simulink model "CusakisME4901delay"  (R2013a)
settings: Solver=ode4  StartTime=0.0  StopTime=inf  FixedStep=0.01  RelTol=1e-3
InitFcn:
  | start_EEVSCube2
  | 
  | %links masses
  | 
  | m=20;%Kg
  | 
  | l=1;%meter
  | 
  | w=0.08;
  | 
  | I=(1/12)*m*(l^2); %moment of inertia
  | 
  | %estimation error
  | 
  | mn=20+m*0.05;
  | In=I+I*0.1;
  | 
  | %controls
  | 
  | a=0.7; %singularity positive gain
  | 
  | %Chaser
  | mb=100;%kg
  | lc=2;%meters
  | lb=lc/2;%meter distance 1joint to CM
  | Ib=(1/12)*mb*(lc^2+lc^2);
  | 
  | %Target
  | 
  | mt=750;%kg target mass
  | lt=1;%meter  side lenght
  | It=(1/6)*(lt^2)*mt;
  | 
  | %Target Initial Conitions
  | 
  | x_t=2;
  | y_t=2;
  | theta_t=0.7853;
  | 
  | Init_t=[x_t;y_t;theta_t;0;0;0];
  | Iinv=pinv(eye(3)*It);
StopFcn:
  | figure(1)
  | subplot(2,1,1)
  | hold on
  | plot(time,kinetic,'g')
  | grid on
  | title('Kinetic Energy vs Time')
  | xlabel('Time')
  | ylabel('Kinetic Energy')
  | hold off
  | 
  | subplot(2,1,2)
  | hold on
  | plot(time,power,'g')
  | grid on
  | title('Power Consumption vs Time')
  | xlabel('Time')
  | ylabel('Power')
  | hold off
  | 
  | chasermapping=[-1,1;-1,-1;1,-1;1,1;-1,1];
  | targetmapping=[1.293,2;2,2.707;2.707,2;2,1.293;1.293,2];
  | 
  | figure(3)
  | hold on
  | plot(EEstate(:,1),EEstate(:,2),'g')
  | plot(targetmapping(:,1),targetmapping(:,2),'r')
  | plot(chasermapping(:,1),chasermapping(:,2),'b')
  | grid on
  | title('End Effector Path')
  | xlabel('X Axis (m)')
  | ylabel('Y Axis (m)')
  | hold off
  | 
  | 
  | figure(4)
  | subplot(2,1,1)
  | hold on
  | plot(time,qqd(:,1),'g')
  | plot(time,qqd(:,2),'r')
  | plot(time,qqd(:,3),'b')
  | grid on
  | title('Theta vs Time')
  | xlabel('Time (sec)')
  | ylabel('Theta (rad)')
  | legend( 'Theta1 ' , ' Theta2 ' , ' Theta3')
  | hold off
  | 
  | subplot(2,1,2)
  | hold on
  | plot(time,qqd(:,4),'g')
  | plot(time,qqd(:,5),'r')
  | plot(time,qqd(:,6),'b')
  | grid on
  | legend( 'Omega1 ' , ' Omega2 ', ' Omega3 ' )
  | title('Omega vs Time')
  | xlabel('Time (sec)')
  | ylabel('Omega (rad/s)')
undefined symbols (not defined in the file): mesh_A, mesh_B, serial
libraries: instrumentlib x5, simulink x3, vrlib x2, dspinverses x1, aerolibanimutils x1
(part 3 of 4)

== matlab function CusakisME4901delay/Differential Kinematics1/Differential Kinematics and singularity avoidance ==
  data: Ve input; qqd input; qd_req output; qd_reqW output; l parameter; a parameter; W output; EE input
function [qd_req,qd_reqW,W]   = fcn( Ve,qqd, l, a,EE)
%Singularity trigger, Alessio Grompone 2013

%computes the Jacobian of a redundant 3R manipulator (end-effector position
%only)measures the rank and gives an error if the rank is < than the number of
%variables

q=[qqd(7) qqd(8) qqd(9)];

%Jacobian position only

Ja=[-(l*sin(q(1))+l*sin(q(1)+q(2))+l*sin(q(1)+q(2)+q(3))) -(l*sin(q(1)+q(2))+l*sin(q(1)+q(2)+q(3))) -l*sin(q(1)+q(2)+q(3));
l*cos(q(1))+l*cos(q(1)+q(2))+l*cos(q(1)+q(2)+q(3)) l*cos(q(1)+q(2))+l*cos(q(1)+q(2)+q(3)) l*cos(q(1)+q(2)+q(3))];

DDD=det(Ja*Ja');
%     %Singularity Measure
% 
W=sqrt(DDD);
if q(2)==0
    
    DW=[0;0;0];
else
%Derivative of the singularity measure obtained in symbolic form
    DW=[                                                                                                                                                                                                                                                                                                                                                                                                                                                                                                                                                                                                                                                                                                                                                                                                                                                                                                                                                                                                                                                                                                                                                                                                                                                                                                                                                                                                                                                                                                                                                                                                                                                                                                                                                                                                                                                                                                                                                                                                                                                                                                                                                                                                                                                                                                                                                                                                                                                                                                                                                                                                                                                                                                                                                                                                                                                                                                                                                                                                                                                                                                                                                                                                                                                                                                                                                                                                                                                                                                                                                                                                                                                                                                                                                                                                                                                                                                                                                                                                                                                                                                                                                                                                                                                                                                                                                                                                                                                                                                                                                                                                                                                                                                                                                                                                                                                                                                                                                                                                                                                                                                                                                                                                                                                                                                                                                                                                                                                                                                                                                                                                                                                                                                                                                                                  0;
                                                                                                                                                                                                                                                                                                                                                                                                                 -(cos(q(1) + q(2) + q(3))*cos(conj(q(1)) + conj(q(2)) + conj(q(3)))*sin(conj(q(1)) + conj(q(2)))*cos(q(1)) - cos(q(1) + q(2) + q(3))*sin(conj(q(1)) + conj(q(2)) + conj(q(3)))*cos(conj(q(1)) + conj(q(2)))*cos(q(1)) + cos(q(1) + q(2) + q(3))*sin(conj(q(1)))*sin(conj(q(1)) + conj(q(2)))*sin(q(1)) - sin(q(1) + q(2) + q(3))*cos(conj(q(1)))*sin(conj(q(1)) + conj(q(2)))*sin(q(1)) + sin(q(1) + q(2) + q(3))*sin(conj(q(1)))*cos(conj(q(1)) + conj(q(2)))*sin(q(1)) - sin(q(1) + q(2) + q(3))*sin(conj(q(1)))*sin(conj(q(1)) + conj(q(2)))*cos(q(1)) + sin(q(1) + q(2) + q(3))*cos(conj(q(1)) + conj(q(2)) + conj(q(3)))*sin(conj(q(1)) + conj(q(2)))*sin(q(1)) - sin(q(1) + q(2) + q(3))*sin(conj(q(1)) + conj(q(2)) + conj(q(3)))*cos(conj(q(1)) + conj(q(2)))*sin(q(1)) + cos(conj(q(1)))*cos(conj(q(1)) + conj(q(2)) + conj(q(3)))*cos(q(1) + q(2))*sin(q(1)) - cos(conj(q(1)))*cos(conj(q(1)) + conj(q(2)) + conj(q(3)))*sin(q(1) + q(2))*cos(q(1)) - cos(conj(q(1)))*sin(conj(q(1)) + conj(q(2)) + conj(q(3)))*cos(q(1) + q(2))*cos(q(1)) + cos(conj(q(1)) + conj(q(2)) + conj(q(3)))*sin(conj(q(1)))*cos(q(1) + q(2))*cos(q(1)) - cos(conj(q(1)))*sin(conj(q(1)) + conj(q(2)) + conj(q(3)))*sin(q(1) + q(2))*sin(q(1)) + cos(conj(q(1)) + conj(q(2)) + conj(q(3)))*sin(conj(q(1)))*sin(q(1) + q(2))*sin(q(1)) + sin(conj(q(1)))*sin(conj(q(1)) + conj(q(2)) + conj(q(3)))*cos(q(1) + q(2))*sin(q(1)) - sin(conj(q(1)))*sin(conj(q(1)) + conj(q(2)) + conj(q(3)))*sin(q(1) + q(2))*cos(q(1)) + cos(conj(q(1)))*cos(conj(q(1)) + conj(q(2)))*cos(q(1) + q(2))*sin(q(1)) - cos(conj(q(1)))*cos(conj(q(1)) + conj(q(2)))*sin(q(1) + q(2))*cos(q(1)) - cos(conj(q(1)))*sin(conj(q(1)) + conj(q(2)))*cos(q(1) + q(2))*cos(q(1)) + sin(conj(q(1)))*cos(conj(q(1)) + conj(q(2)))*cos(q(1) + q(2))*cos(q(1)) + cos(q(1) + q(2) + q(3))*cos(conj(q(1)))*cos(conj(q(1)) + conj(q(2)) + conj(q(3)))*sin(q(1) + q(2)) - sin(q(1) + q(2) + q(3))*cos(conj(q(1)))*cos(conj(q(1)) + conj(q(2)) + conj(q(3)))*cos(q(1) + q(2)) - cos(conj(q(1)))*sin(conj(q(1)) + conj(q(2)))*sin(q(1) + q(2))*sin(q(1)) + sin(conj(q(1)))*cos(conj(q(1)) + conj(q(2)))*sin(q(1) + q(2))*sin(q(1)) + sin(conj(q(1)))*sin(conj(q(1)) + conj(q(2)))*cos(q(1) + q(2))*sin(q(1)) - sin(conj(q(1)))*sin(conj(q(1)) + conj(q(2)))*sin(q(1) + q(2))*cos(q(1)) + cos(q(1) + q(2) + q(3))*sin(conj(q(1)))*sin(conj(q(1)) + conj(q(2)) + conj(q(3)))*sin(q(1) + q(2)) - sin(q(1) + q(2) + q(3))*sin(conj(q(1)))*sin(conj(q(1)) + conj(q(2)) + conj(q(3)))*cos(q(1) + q(2)) + 2*cos(q(1) + q(2) + q(3))*cos(conj(q(1)))*cos(conj(q(1)) + conj(q(2)) + conj(q(3)))*sin(q(1)) - 2*cos(q(1) + q(2) + q(3))*cos(conj(q(1)))*sin(conj(q(1)) + conj(q(2)) + conj(q(3)))*cos(q(1)) + 2*cos(q(1) + q(2) + q(3))*cos(conj(q(1)) + conj(q(2)) + conj(q(3)))*sin(conj(q(1)))*cos(q(1)) - 2*sin(q(1) + q(2) + q(3))*cos(conj(q(1)))*cos(conj(q(1)) + conj(q(2)) + conj(q(3)))*cos(q(1)) + 2*cos(q(1) + q(2) + q(3))*sin(conj(q(1)))*sin(conj(q(1)) + conj(q(2)) + conj(q(3)))*sin(q(1)) - 2*sin(q(1) + q(2) + q(3))*cos(conj(q(1)))*sin(conj(q(1)) + conj(q(2)) + conj(q(3)))*sin(q(1)) + 2*sin(q(1) + q(2) + q(3))*cos(conj(q(1)) + conj(q(2)) + conj(q(3)))*sin(conj(q(1)))*sin(q(1)) - 2*sin(q(1) + q(2) + q(3))*sin(conj(q(1)))*sin(conj(q(1)) + conj(q(2)) + conj(q(3)))*cos(q(1)) + cos(q(1) + q(2) + q(3))*cos(conj(q(1)))*cos(conj(q(1)) + conj(q(2)))*sin(q(1)) - cos(q(1) + q(2) + q(3))*cos(conj(q(1)))*sin(conj(q(1)) + conj(q(2)))*cos(q(1)) + cos(q(1) + q(2) + q(3))*sin(conj(q(1)))*cos(conj(q(1)) + conj(q(2)))*cos(q(1)) - sin(q(1) + q(2) + q(3))*cos(conj(q(1)))*cos(conj(q(1)) + conj(q(2)))*cos(q(1)))/(2*(cos(q(1) + q(2) + q(3))*sin(conj(q(1)))*cos(conj(q(1)) + conj(q(2)))*sin(q(1)) - cos(q(1) + q(2) + q(3))*cos(conj(q(1)))*sin(conj(q(1)) + conj(q(2)))*sin(q(1)) + sin(q(1) + q(2) + q(3))*cos(conj(q(1)))*sin(conj(q(1)) + conj(q(2)))*cos(q(1)) - sin(q(1) + q(2) + q(3))*sin(conj(q(1)))*cos(conj(q(1)) + conj(q(2)))*cos(q(1)) + cos(q(1) + q(2) + q(3))*cos(conj(q(1)) + conj(q(2)) + conj(q(3)))*sin(conj(q(1)) + conj(q(2)))*sin(q(1)) - cos(q(1) + q(2) + q(3))*sin(conj(q(1)) + conj(q(2)) + conj(q(3)))*cos(conj(q(1)) + conj(q(2)))*sin(q(1)) - sin(q(1) + q(2) + q(3))*cos(conj(q(1)) + conj(q(2)) + conj(q(3)))*sin(conj(q(1)) + conj(q(2)))*cos(q(1)) + sin(q(1) + q(2) + q(3))*sin(conj(q(1)) + conj(q(2)) + conj(q(3)))*cos(conj(q(1)) + conj(q(2)))*cos(q(1)) - cos(conj(q(1)))*sin(conj(q(1)) + conj(q(2)) + conj(q(3)))*cos(q(1) + q(2))*sin(q(1)) + cos(conj(q(1)))*sin(conj(q(1)) + conj(q(2)) + conj(q(3)))*sin(q(1) + q(2))*cos(q(1)) + cos(conj(q(1)) + conj(q(2)) + conj(q(3)))*sin(conj(q(1)))*cos(q(1) + q(2))*sin(q(1)) - cos(conj(q(1)) + conj(q(2)) + conj(q(3)))*sin(conj(q(1)))*sin(q(1) + q(2))*cos(q(1)) - cos(conj(q(1)))*sin(conj(q(1)) + conj(q(2)))*cos(q(1) + q(2))*sin(q(1)) + cos(conj(q(1)))*sin(conj(q(1)) + conj(q(2)))*sin(q(1) + q(2))*cos(q(1)) + sin(conj(q(1)))*cos(conj(q(1)) + conj(q(2)))*cos(q(1) + q(2))*sin(q(1)) - sin(conj(q(1)))*cos(conj(q(1)) + conj(q(2)))*sin(q(1) + q(2))*cos(q(1)) - cos(q(1) + q(2) + q(3))*cos(conj(q(1)))*sin(conj(q(1)) + conj(q(2)) + conj(q(3)))*sin(q(1) + q(2)) + cos(q(1) + q(2) + q(3))*cos(conj(q(1)) + conj(q(2)) + conj(q(3)))*sin(conj(q(1)))*sin(q(1) + q(2)) + sin(q(1) + q(2) + q(3))*cos(conj(q(1)))*sin(conj(q(1)) + conj(q(2)) + conj(q(3)))*cos(q(1) + q(2)) - sin(q(1) + q(2) + q(3))*cos(conj(q(1)) + conj(q(2)) + conj(q(3)))*sin(conj(q(1)))*cos(q(1) + q(2)) - 2*cos(q(1) + q(2) + q(3))*cos(conj(q(1)))*sin(conj(q(1)) + conj(q(2)) + conj(q(3)))*sin(q(1)) + 2*cos(q(1) + q(2) + q(3))*cos(conj(q(1)) + conj(q(2)) + conj(q(3)))*sin(conj(q(1)))*sin(q(1)) + 2*sin(q(1) + q(2) + q(3))*cos(conj(q(1)))*sin(conj(q(1)) + conj(q(2)) + conj(q(3)))*cos(q(1)) - 2*sin(q(1) + q(2) + q(3))*cos(conj(q(1)) + conj(q(2)) + conj(q(3)))*sin(conj(q(1)))*cos(q(1)) + 2*cos(q(1) + q(2) + q(3))*cos(conj(q(1)) + conj(q(2)) + conj(q(3)))*sin(conj(q(1)) + conj(q(2)))*sin(q(1) + q(2)) - 2*cos(q(1) + q(2) + q(3))*sin(conj(q(1)) + conj(q(2)) + conj(q(3)))*cos(conj(q(1)) + conj(q(2)))*sin(q(1) + q(2)) - 2*sin(q(1) + q(2) + q(3))*cos(conj(q(1)) + conj(q(2)) + conj(q(3)))*sin(conj(q(1)) + conj(q(2)))*cos(q(1) + q(2)) + 2*sin(q(1) + q(2) + q(3))*sin(conj(q(1)) + conj(q(2)) + conj(q(3)))*cos(conj(q(1)) + conj(q(2)))*cos(q(1) + q(2)))^(1/2));
 -(cos(q(1) + q(2) + q(3))*cos(conj(q(1)) + conj(q(2)) + conj(q(3)))*cos(conj(q(1)) + conj(q(2)))*sin(q(1)) + cos(q(1) + q(2) + q(3))*cos(conj(q(1)) + conj(q(2)) + conj(q(3)))*sin(conj(q(1)) + conj(q(2)))*cos(q(1)) - cos(q(1) + q(2) + q(3))*sin(conj(q(1)) + conj(q(2)) + conj(q(3)))*cos(conj(q(1)) + conj(q(2)))*cos(q(1)) - sin(q(1) + q(2) + q(3))*cos(conj(q(1)) + conj(q(2)) + conj(q(3)))*cos(conj(q(1)) + conj(q(2)))*cos(q(1)) - sin(q(1) + q(2) + q(3))*cos(conj(q(1)))*sin(conj(q(1)) + conj(q(2)))*sin(q(1)) + sin(q(1) + q(2) + q(3))*sin(conj(q(1)))*cos(conj(q(1)) + conj(q(2)))*sin(q(1)) + cos(q(1) + q(2) + q(3))*sin(conj(q(1)) + conj(q(2)) + conj(q(3)))*sin(conj(q(1)) + conj(q(2)))*sin(q(1)) + sin(q(1) + q(2) + q(3))*cos(conj(q(1)) + conj(q(2)) + conj(q(3)))*sin(conj(q(1)) + conj(q(2)))*sin(q(1)) - sin(q(1) + q(2) + q(3))*sin(conj(q(1)) + conj(q(2)) + conj(q(3)))*cos(conj(q(1)) + conj(q(2)))*sin(q(1)) - sin(q(1) + q(2) + q(3))*sin(conj(q(1)) + conj(q(2)) + conj(q(3)))*sin(conj(q(1)) + conj(q(2)))*cos(q(1)) + cos(conj(q(1)))*cos(conj(q(1)) + conj(q(2)) + conj(q(3)))*cos(q(1) + q(2))*sin(q(1)) - cos(conj(q(1)))*cos(conj(q(1)) + conj(q(2)) + conj(q(3)))*sin(q(1) + q(2))*cos(q(1)) + sin(conj(q(1)))*sin(conj(q(1)) + conj(q(2)) + conj(q(3)))*cos(q(1) + q(2))*sin(q(1)) - sin(conj(q(1)))*sin(conj(q(1)) + conj(q(2)) + conj(q(3)))*sin(q(1) + q(2))*cos(q(1)) + cos(q(1) + q(2) + q(3))*cos(conj(q(1)))*cos(conj(q(1)) + conj(q(2)) + conj(q(3)))*sin(q(1) + q(2)) - cos(q(1) + q(2) + q(3))*cos(conj(q(1)))*sin(conj(q(1)) + conj(q(2)) + conj(q(3)))*cos(q(1) + q(2)) + cos(q(1) + q(2) + q(3))*cos(conj(q(1)) + conj(q(2)) + conj(q(3)))*sin(conj(q(1)))*cos(q(1) + q(2)) - sin(q(1) + q(2) + q(3))*cos(conj(q(1)))*cos(conj(q(1)) + conj(q(2)) + conj(q(3)))*cos(q(1) + q(2)) + cos(q(1) + q(2) + q(3))*sin(conj(q(1)))*sin(conj(q(1)) + conj(q(2)) + conj(q(3)))*sin(q(1) + q(2)) - sin(q(1) + q(2) + q(3))*cos(conj(q(1)))*sin(conj(q(1)) + conj(q(2)) + conj(q(3)))*sin(q(1) + q(2)) + sin(q(1) + q(2) + q(3))*cos(conj(q(1)) + conj(q(2)) + conj(q(3)))*sin(conj(q(1)))*sin(q(1) + q(2)) - sin(q(1) + q(2) + q(3))*sin(conj(q(1)))*sin(conj(q(1)) + conj(q(2)) + conj(q(3)))*cos(q(1) + q(2)) + 2*cos(q(1) + q(2) + q(3))*cos(conj(q(1)))*cos(conj(q(1)) + conj(q(2)) + conj(q(3)))*sin(q(1)) - 2*cos(q(1) + q(2) + q(3))*cos(conj(q(1)))*sin(conj(q(1)) + conj(q(2)) + conj(q(3)))*cos(q(1)) + 2*cos(q(1) + q(2) + q(3))*cos(conj(q(1)) + conj(q(2)) + conj(q(3)))*sin(conj(q(1)))*cos(q(1)) - 2*sin(q(1) + q(2) + q(3))*cos(conj(q(1)))*cos(conj(q(1)) + conj(q(2)) + conj(q(3)))*cos(q(1)) + 2*cos(q(1) + q(2) + q(3))*cos(conj(q(1)) + conj(q(2)) + conj(q(3)))*cos(conj(q(1)) + conj(q(2)))*sin(q(1) + q(2)) + 2*cos(q(1) + q(2) + q(3))*cos(conj(q(1)) + conj(q(2)) + conj(q(3)))*sin(conj(q(1)) + conj(q(2)))*cos(q(1) + q(2)) - 2*cos(q(1) + q(2) + q(3))*sin(conj(q(1)) + conj(q(2)) + conj(q(3)))*cos(conj(q(1)) + conj(q(2)))*cos(q(1) + q(2)) - 2*sin(q(1) + q(2) + q(3))*cos(conj(q(1)) + conj(q(2)) + conj(q(3)))*cos(conj(q(1)) + conj(q(2)))*cos(q(1) + q(2)) + 2*cos(q(1) + q(2) + q(3))*sin(conj(q(1)))*sin(conj(q(1)) + conj(q(2)) + conj(q(3)))*sin(q(1)) - 2*sin(q(1) + q(2) + q(3))*cos(conj(q(1)))*sin(conj(q(1)) + conj(q(2)) + conj(q(3)))*sin(q(1)) + 2*sin(q(1) + q(2) + q(3))*cos(conj(q(1)) + conj(q(2)) + conj(q(3)))*sin(conj(q(1)))*sin(q(1)) - 2*sin(q(1) + q(2) + q(3))*sin(conj(q(1)))*sin(conj(q(1)) + conj(q(2)) + conj(q(3)))*cos(q(1)) + 2*cos(q(1) + q(2) + q(3))*sin(conj(q(1)) + conj(q(2)) + conj(q(3)))*sin(conj(q(1)) + conj(q(2)))*sin(q(1) + q(2)) + 2*sin(q(1) + q(2) + q(3))*cos(conj(q(1)) + conj(q(2)) + conj(q(3)))*sin(conj(q(1)) + conj(q(2)))*sin(q(1) + q(2)) - 2*sin(q(1) + q(2) + q(3))*sin(conj(q(1)) + conj(q(2)) + conj(q(3)))*cos(conj(q(1)) + conj(q(2)))*sin(q(1) + q(2)) - 2*sin(q(1) + q(2) + q(3))*sin(conj(q(1)) + conj(q(2)) + conj(q(3)))*sin(conj(q(1)) + conj(q(2)))*cos(q(1) + q(2)) - cos(q(1) + q(2) + q(3))*cos(conj(q(1)))*sin(conj(q(1)) + conj(q(2)))*cos(q(1)) + cos(q(1) + q(2) + q(3))*sin(conj(q(1)))*cos(conj(q(1)) + conj(q(2)))*cos(q(1)))/(2*(cos(q(1) + q(2) + q(3))*sin(conj(q(1)))*cos(conj(q(1)) + conj(q(2)))*sin(q(1)) - cos(q(1) + q(2) + q(3))*cos(conj(q(1)))*sin(conj(q(1)) + conj(q(2)))*sin(q(1)) + sin(q(1) + q(2) + q(3))*cos(conj(q(1)))*sin(conj(q(1)) + conj(q(2)))*cos(q(1)) - sin(q(1) + q(2) + q(3))*sin(conj(q(1)))*cos(conj(q(1)) + conj(q(2)))*cos(q(1)) + cos(q(1) + q(2) + q(3))*cos(conj(q(1)) + conj(q(2)) + conj(q(3)))*sin(conj(q(1)) + conj(q(2)))*sin(q(1)) - cos(q(1) + q(2) + q(3))*sin(conj(q(1)) + conj(q(2)) + conj(q(3)))*cos(conj(q(1)) + conj(q(2)))*sin(q(1)) - sin(q(1) + q(2) + q(3))*cos(conj(q(1)) + conj(q(2)) + conj(q(3)))*sin(conj(q(1)) + conj(q(2)))*cos(q(1)) + sin(q(1) + q(2) + q(3))*sin(conj(q(1)) + conj(q(2)) + conj(q(3)))*cos(conj(q(1)) + conj(q(2)))*cos(q(1)) - cos(conj(q(1)))*sin(conj(q(1)) + conj(q(2)) + conj(q(3)))*cos(q(1) + q(2))*sin(q(1)) + cos(conj(q(1)))*sin(conj(q(1)) + conj(q(2)) + conj(q(3)))*sin(q(1) + q(2))*cos(q(1)) + cos(conj(q(1)) + conj(q(2)) + conj(q(3)))*sin(conj(q(1)))*cos(q(1) + q(2))*sin(q(1)) - cos(conj(q(1)) + conj(q(2)) + conj(q(3)))*sin(conj(q(1)))*sin(q(1) + q(2))*cos(q(1)) - cos(conj(q(1)))*sin(conj(q(1)) + conj(q(2)))*cos(q(1) + q(2))*sin(q(1)) + cos(conj(q(1)))*sin(conj(q(1)) + conj(q(2)))*sin(q(1) + q(2))*cos(q(1)) + sin(conj(q(1)))*cos(conj(q(1)) + conj(q(2)))*cos(q(1) + q(2))*sin(q(1)) - sin(conj(q(1)))*cos(conj(q(1)) + conj(q(2)))*sin(q(1) + q(2))*cos(q(1)) - cos(q(1) + q(2) + q(3))*cos(conj(q(1)))*sin(conj(q(1)) + conj(q(2)) + conj(q(3)))*sin(q(1) + q(2)) + cos(q(1) + q(2) + q(3))*cos(conj(q(1)) + conj(q(2)) + conj(q(3)))*sin(conj(q(1)))*sin(q(1) + q(2)) + sin(q(1) + q(2) + q(3))*cos(conj(q(1)))*sin(conj(q(1)) + conj(q(2)) + conj(q(3)))*cos(q(1) + q(2)) - sin(q(1) + q(2) + q(3))*cos(conj(q(1)) + conj(q(2)) + conj(q(3)))*sin(conj(q(1)))*cos(q(1) + q(2)) - 2*cos(q(1) + q(2) + q(3))*cos(conj(q(1)))*sin(conj(q(1)) + conj(q(2)) + conj(q(3)))*sin(q(1)) + 2*cos(q(1) + q(2) + q(3))*cos(conj(q(1)) + conj(q(2)) + conj(q(3)))*sin(conj(q(1)))*sin(q(1)) + 2*sin(q(1) + q(2) + q(3))*cos(conj(q(1)))*sin(conj(q(1)) + conj(q(2)) + conj(q(3)))*cos(q(1)) - 2*sin(q(1) + q(2) + q(3))*cos(conj(q(1)) + conj(q(2)) + conj(q(3)))*sin(conj(q(1)))*cos(q(1)) + 2*cos(q(1) + q(2) + q(3))*cos(conj(q(1)) + conj(q(2)) + conj(q(3)))*sin(conj(q(1)) + conj(q(2)))*sin(q(1) + q(2)) - 2*cos(q(1) + q(2) + q(3))*sin(conj(q(1)) + conj(q(2)) + conj(q(3)))*cos(conj(q(1)) + conj(q(2)))*sin(q(1) + q(2)) - 2*sin(q(1) + q(2) + q(3))*cos(conj(q(1)) + conj(q(2)) + conj(q(3)))*sin(conj(q(1)) + conj(q(2)))*cos(q(1) + q(2)) + 2*sin(q(1) + q(2) + q(3))*sin(conj(q(1)) + conj(q(2)) + conj(q(3)))*cos(conj(q(1)) + conj(q(2)))*cos(q(1) + q(2)))^(1/2))];
end
Jinv=pinv(Ja); %inverse of the Jacobian

qa=a*DW;

qd_req=Jinv*Ve;
%qd_reqW=Jinv*Ve+(eye(3)-Jinv*Ja)*qa;%With singularity avoidance
EEv=[0;0;EE];
qd_req(3)=qd_req(3)+EE;
%qd_reqW(3)=qd_reqW(3)+EE;
% 

Jstar=Ja;
A=svd(Jstar);
lambmax=20;
Sigma=A(2);
if Sigma>=0.5 
lamb2=0;
else
lamb2=(1-((Sigma)/4)^2)*lambmax;
end
qd_reqW=(Jstar'*pinv(Jstar*Jstar'+(lamb2)*eye(2)))*Ve+EEv;





end

== matlab function CusakisME4901delay/GamePad Input/MATLAB Function ==
  data: u output; but output; Axes input; Buttons input; j output
function [u,but,j]  = fcn(Axes,Buttons)
%#Mapping buttons for KRAUN Gamepad
%Alessio Grompone

%%%%%%%%%%%%%%%%%%%%%%%%%%%%%%%%%%%%%%%%%%%%%%%%%%%%
%       Home Gamepad
%Axes

if Axes(2)==-1
    %Up
    u=[1;0];
elseif Axes(2)==1
        %Down
    u=[-1;0];   
elseif  Axes(1)==-1
    %Left
    u=[0;1];
elseif  Axes(1)==1 
    %Right
    u=[0;-1];
else
    %NO Axes Command
    u=[0;0];
end

if Buttons(5)==1
j=1;
else
if Buttons(6)==1
    j=-1;
else
    j=0;
end
end

if Buttons(1)==1
    %Button1
    but=[1;0;0;0];
elseif Buttons(2)==1
    %Button1
    but=[0;1;0;0];
elseif Buttons(3)==1
    %Button1
    but=[0;0;1;0];
elseif Buttons(4)==1
    %Button1
    but=[0;0;0;1];
else
    %NO Button command
    but=[0;0;0;0];
end
end

== matlab function CusakisME4901delay/Collision/Collision/Collision ==
  data: epsilon input; dock_sensA_c output; dock_sensB_c output; n_c output; QA_c output; QB_c output; sigma_dock input; dotsigma_dock input; Rbi_A1 input; Rbi_B1 input; A output; B output; Xcm_A input; Xcm_B input; mesh_A input; mesh_B input; dock_sensA input; dock_sensB input; sigma input; docking output; ma_mb_Ia_Ib input; collision output; Vcm_an output; Vcm_bn output; W_an output; W_bn output; j output
function [dock_sensA_c,dock_sensB_c,n_c,QA_c,QB_c,A,B,docking,collision,Vcm_an,Vcm_bn,W_an,W_bn,j] = fcn(epsilon,sigma_dock,dotsigma_dock,Rbi_A1,Rbi_B1,Xcm_A,Xcm_B,mesh_A,mesh_B,dock_sensA,dock_sensB,sigma,ma_mb_Ia_Ib)

[dock_sensA_c,dock_sensB_c,n_c,QA_c,QB_c,A,B,docking,collision,Vcm_an,Vcm_bn,W_an,W_bn,j] = collision_function(epsilon,sigma_dock,dotsigma_dock,Rbi_A1,Rbi_B1,Xcm_A,Xcm_B,mesh_A,mesh_B,dock_sensA,dock_sensB,sigma,ma_mb_Ia_Ib);

== matlab function CusakisME4901delay/Collision/Collision/Embedded MATLAB Function10 ==
  data: M input; DD output
function DD=fcn(M)

[m,n] = size(M);
a = zeros(n*m,1);
MM=zeros(n*m,1);
i=1;
for mm=0:m:n*m-1
for j=1:1:m
    a(j+mm,1)=M(j,i); 
end
i=i+1;
end
DD=a;

== matlab function CusakisME4901delay/Collision/Collision/Embedded MATLAB Function9 ==
  data: M input; DD output
function DD=fcn(M)

[m,n] = size(M);
a = zeros(n*m,1);
MM=zeros(n*m,1);
i=1;
for mm=0:m:n*m-1
for j=1:1:m
    a(j+mm,1)=M(j,i); 
end
i=i+1;
end
DD=a;

== matlab function CusakisME4901delay/Collision/Dynamics/MATLAB Function ==
  data: u input; y output; ur input; coll input
function y = fcn(u,ur,coll)
%#codegen



if coll==0 

y = ur;

else 
    
y=u;
    
end

== matlab function CusakisME4901delay/Collision/StateVectormapping/Rotation MAtrix1 ==
  data: u input; y output; R output
function [y,R] = fcn(u)
%#codegen

y=[u(1);u(2); 0; u(4); u(5); 0; 0; 0; u(6)];



R = [cos(u(3)) -sin(u(3));
    sin(u(3)) cos(u(3))];

end

== matlab function CusakisME4901delay/Differential Kinematics1/3rd link Kinematics ==
  data: qqd input; SC input; dSC input; state_3link output; lb parameter; l parameter; EE output; mb parameter; m parameter; Rcm output
function [state_3link,EE,Rcm] = fcn(qqd,SC,dSC,lb,l,mb,m)
%#codegen

%fixed base position

xb=SC(1);
yb=SC(2);
thetab=SC(6);
thetabb=dSC(6);


%state vector of the third link
state_3link=zeros([6,1]);

state_3link(1)=xb+lb*cos(thetab)+l*cos(qqd(7)+thetab)+l*cos(qqd(8)+qqd(7)+thetab)+(l/2)*cos(qqd(9)+qqd(8)+qqd(7)+thetab);%X inertia position of the CM of the third Link
state_3link(2)=yb+lb*sin(thetab)+l*sin(qqd(7)+thetab)+l*sin(qqd(8)+qqd(7)+thetab)+(l/2)*sin(qqd(9)+qqd(8)+qqd(7)+thetab);%Y inertia position of the CM of the third Link
state_3link(3)=qqd(9)+qqd(8)+qqd(7)+thetab;%theta inertia position of the CM of the third Link
state_3link(4)=-lb*thetabb*sin(thetab)-l*(qqd(4)+thetabb)*sin(qqd(7)+thetab)-l*(qqd(4)+qqd(5)+thetabb)*sin(qqd(8)+qqd(7)+thetab)-(l/2)*(qqd(4)+qqd(5)+qqd(6)+thetabb)*sin(qqd(9)+qqd(8)+qqd(7)+thetab);%VX inertia position of the CM of the third Link
state_3link(5)=lb*thetabb*cos(thetab)+l*(qqd(4)+thetabb)*cos(qqd(7)+thetab)+l*(qqd(4)+qqd(5)+thetabb)*cos(qqd(8)+qqd(7)+thetab)+(l/2)*(qqd(4)+qqd(5)+qqd(6)+thetabb)*cos(qqd(9)+qqd(8)+qqd(7)+thetab);%VY inertia position of the CM of the third Link;%X inertia position of the CM of the third Link
state_3link(6)=qqd(4)+qqd(5)+qqd(6)+thetabb;%omega inertia position of the CM of the third Link

%end effector position inertia frame
EE=zeros([6,1]);

EE(1)=xb+lb*cos(thetab)+l*cos(qqd(7)+thetab)+l*cos(qqd(8)+qqd(7)+thetab)+(l)*cos(qqd(9)+qqd(8)+qqd(7)+thetab);%X inertia position of the CM of the third Link
EE(2)=yb+lb*sin(thetab)+l*sin(qqd(7)+thetab)+l*sin(qqd(8)+qqd(7)+thetab)+(l)*sin(qqd(9)+qqd(8)+qqd(7)+thetab);%Y inertia position of the CM of the third Link
EE(3)=qqd(9)+qqd(8)+qqd(7)+thetab;%theta inertia position of the CM of the third Link
EE(4)=-lb*thetabb*sin(thetab)-l*(qqd(4)+thetabb)*sin(qqd(7)+thetab)-l*(qqd(4)+qqd(5)+thetabb)*sin(qqd(8)+qqd(7)+thetab)-(l)*(qqd(4)+qqd(5)+qqd(6)+thetabb)*sin(qqd(9)+qqd(8)+qqd(7)+thetab);%VX inertia position of the CM of the third Link
EE(5)=lb*thetabb*cos(thetab)+l*(qqd(4)+thetabb)*cos(qqd(7)+thetab)+l*(qqd(4)+qqd(5)+thetabb)*cos(qqd(8)+qqd(7)+thetab)+(l)*(qqd(4)+qqd(5)+qqd(6)+thetabb)*cos(qqd(9)+qqd(8)+qqd(7)+thetab);%VY inertia position of the CM of the third Link;%X inertia position of the CM of the third Link
EE(6)=qqd(4)+qqd(5)+qqd(6)+thetabb;%omega inertia position of the CM of the third Link



M=m*3+mb;%total mass

r0=[xb;yb;0];


V=[qqd(7) qqd(4) qqd(1) qqd(8) qqd(5) qqd(2) qqd(9) qqd(6) qqd(3) thetab thetabb 0];

%joints to joint position vectors 
pl1=[lb*cos(V(10));lb*sin(V(10));0];
pl2=[l*cos(V(1)+V(10));l*sin(V(1)+V(10));0];
pl3=[l*cos(V(1)+V(4)+V(10));l*sin(V(1)+V(4)+V(10));0];
%joint3 to EndEffector position vectors 
plr=[l*cos(V(1)+V(4)+V(7)+V(10));
    l*sin(V(1)+V(4)+V(7)+V(10));0];

%Position Vectors of each Joint
p1=r0+pl1;
p2=r0+pl1+pl2;
p3=r0+pl1+pl2+pl3;

%Position Vector CM of each link
r1=p1+[(l/2)*cos(V(1)+V(10));(l/2)*sin(V(1)+V(10));0];
r2=p2+[(l/2)*cos(V(1)+V(4)+V(10));(l/2)*sin(V(1)+V(4)+V(10));0];
r3=p3+[(l/2)*cos(V(1)+V(4)+V(7)+V(10));(l/2)*sin(V(1)+V(4)+V(7)+V(10));0];

%CM position inertia frame
rg=(mb/M)*r0+(m/M)*(r1+r2+r3);
roc=rg-r0;


%Position Vector of EndEffector
pr=r0+pl1+pl2+pl3+plr;

%distance end effector center of mass (body frame) 
Rcm=roc-pr;
end

== matlab function CusakisME4901delay/Collision/StateVectormapping1/Rotation MAtrix1 ==
  data: u1 input; y output; R output; u2 input; u3 input; u4 input; u5 input; u6 input
function [y,R] = fcn(u1,u2,u3,u4,u5,u6)
%#codegen

% y=[u(1);u(2); 0; u(4); u(5); 0; 0; u(6)];

y=[u1;u2;0;u4;u5;0;0;0;u6];
theta=u3;

R = [cos(theta) -sin(theta);
    sin(theta) cos(theta)];

end

== matlab function CusakisME4901delay/Collision/Dynamics/Initial Position Target ==
  data: u input; i input; y output
function y = fcn(u,i)
%#codegen

y=u+i;

== matlab function CusakisME4901delay/Docking End Simulation/Docking and collision Detection ==
  data: Docking input; Dock_button input; Stop output; Collisn input; Count output; Coll input
function [Stop,Count]   = fcn( Docking, Dock_button,Collisn,Coll)
%Singularity trigger, Alessio Grompone 2013

if Docking==0
    Stop=0;
else
    if Dock_button(1)==1
     Stop=1;
    else
     Stop=0;
    end    
end

if Collisn==1
    Count=1+Coll;
else
    Count=Coll;
end

== matlab function CusakisME4901delay/Energy Measures/MATLAB Function ==
  data: T output; u input; m parameter; l parameter; w parameter
function T  = fcn(u,m,l,w)
%#codegen


theta1=u(1);
theta_dot1=u(2);
theta2=theta1+u(3);
theta_dot2=theta_dot1+u(4);
theta3=theta2+u(5);
theta_dot3=theta_dot2+u(6);




%%%%%%%%%%%%%%%%%%%%%%%%%%%%%%%%%

T=(m*((theta_dot1*l.*sin(theta1) + theta_dot2*l.*sin(theta2) + (theta_dot3*l.*sin(theta3))/2).^2 + (theta_dot1*l.*cos(theta1) + theta_dot2*l.*cos(theta2) + (theta_dot3*l.*cos(theta3))/2).^2))/2 + (m*((theta_dot1*l.*cos(theta1) + (theta_dot2*l.*cos(theta2))/2).^2 + (theta_dot1*l.*sin(theta1) + (theta_dot2*l.*sin(theta2))/2).^2))/2 + (theta_dot1.^2*l^2*m)/8 + (theta_dot1.^2*m*(l^2 + w^2))/24 + (theta_dot2.^2*m*(l^2 + w^2))/24 + (theta_dot3.^2*m*(l^2 + w^2))/24;

== matlab function CusakisME4901delay/Differential Kinematics1/Diff Kinematics ==
  data: qd_req output; qd_reqW output; qqd input; q3rd input; Ve input; SC input; l parameter; m parameter; I parameter; lb parameter; mb parameter; Ib parameter; Jstar output; SCnew output
function [qd_req,qd_reqW,Jstar,SCnew]    = fcn(qqd,q3rd,Ve,SC,l,m,I,lb,mb,Ib)

q1=qqd(7);
q2=qqd(8);
q3=qqd(9);
qd1=qqd(4);
qd2=qqd(5);
qd3=qqd(6);


base_x=SC(1);
base_y=SC(2);
bth=SC(6);
%XU KANADE matrices

Hb=[                                                                                                                                                                       3*m + mb,                                                                                                                                                                             0,                                                                                                                                                                              0,                                                                                                                                                                                                                                                                                                                                                                                                0,                                                                                                                                                                                                                                                                                                                                                                                                0,                                                                                                                                                                                                                                           -(3*m + mb)*((base_y*mb)/(3*m + mb) - base_y + (m*(3*base_y + (l*sin(bth + q1 + q2 + q3))/2 + (5*l*sin(bth + q1))/2 + 3*lb*sin(bth) + (3*l*sin(bth + q1 + q2))/2))/(3*m + mb));
                                                                                                                                                                              0,                                                                                                                                                                      3*m + mb,                                                                                                                                                                              0,                                                                                                                                                                                                                                                                                                                                                                                                0,                                                                                                                                                                                                                                                                                                                                                                                                0,                                                                                                                                                                                                                                            (3*m + mb)*((base_x*mb)/(3*m + mb) - base_x + (m*(3*base_x + (l*cos(bth + q1 + q2 + q3))/2 + (5*l*cos(bth + q1))/2 + 3*lb*cos(bth) + (3*l*cos(bth + q1 + q2))/2))/(3*m + mb));
                                                                                                                                                                              0,                                                                                                                                                                             0,                                                                                                                                                                       3*m + mb,                                                                                                                                                                                                                    (3*m + mb)*((base_y*mb)/(3*m + mb) - base_y + (m*(3*base_y + (l*sin(bth + q1 + q2 + q3))/2 + (5*l*sin(bth + q1))/2 + 3*lb*sin(bth) + (3*l*sin(bth + q1 + q2))/2))/(3*m + mb)),                                                                                                                                                                                                                   -(3*m + mb)*((base_x*mb)/(3*m + mb) - base_x + (m*(3*base_x + (l*cos(bth + q1 + q2 + q3))/2 + (5*l*cos(bth + q1))/2 + 3*lb*cos(bth) + (3*l*cos(bth + q1 + q2))/2))/(3*m + mb)),                                                                                                                                                                                                                                                                                                                                                                                                                        0;
                                                                                                                                                                              0,                                                                                                                                                                             0,  (3*m + mb)*((base_y*mb)/(3*m + mb) - base_y + (m*(3*base_y + (l*sin(bth + q1 + q2 + q3))/2 + (5*l*sin(bth + q1))/2 + 3*lb*sin(bth) + (3*l*sin(bth + q1 + q2))/2))/(3*m + mb)),                                                                                                                                                                                 3*I + Ib + m*(l*sin(bth + q1) + lb*sin(bth) + (l*sin(bth + q1 + q2))/2)^2 + m*((l*sin(bth + q1))/2 + lb*sin(bth))^2 + m*((l*sin(bth + q1 + q2 + q3))/2 + l*sin(bth + q1) + lb*sin(bth) + l*sin(bth + q1 + q2))^2, 3*I + Ib - m*(l*cos(bth + q1) + lb*cos(bth) + (l*cos(bth + q1 + q2))/2)*(l*sin(bth + q1) + lb*sin(bth) + (l*sin(bth + q1 + q2))/2) - m*((l*cos(bth + q1))/2 + lb*cos(bth))*((l*sin(bth + q1))/2 + lb*sin(bth)) - m*((l*cos(bth + q1 + q2 + q3))/2 + l*cos(bth + q1) + lb*cos(bth) + l*cos(bth + q1 + q2))*((l*sin(bth + q1 + q2 + q3))/2 + l*sin(bth + q1) + lb*sin(bth) + l*sin(bth + q1 + q2)),                                                                                                                                                                                                                                                                                                                                                                                                                 3*I + Ib;
                                                                                                                                                                              0,                                                                                                                                                                             0, -(3*m + mb)*((base_x*mb)/(3*m + mb) - base_x + (m*(3*base_x + (l*cos(bth + q1 + q2 + q3))/2 + (5*l*cos(bth + q1))/2 + 3*lb*cos(bth) + (3*l*cos(bth + q1 + q2))/2))/(3*m + mb)), 3*I + Ib - m*(l*cos(bth + q1) + lb*cos(bth) + (l*cos(bth + q1 + q2))/2)*(l*sin(bth + q1) + lb*sin(bth) + (l*sin(bth + q1 + q2))/2) - m*((l*cos(bth + q1))/2 + lb*cos(bth))*((l*sin(bth + q1))/2 + lb*sin(bth)) - m*((l*cos(bth + q1 + q2 + q3))/2 + l*cos(bth + q1) + lb*cos(bth) + l*cos(bth + q1 + q2))*((l*sin(bth + q1 + q2 + q3))/2 + l*sin(bth + q1) + lb*sin(bth) + l*sin(bth + q1 + q2)),                                                                                                                                                                                 3*I + Ib + m*(l*cos(bth + q1) + lb*cos(bth) + (l*cos(bth + q1 + q2))/2)^2 + m*((l*cos(bth + q1))/2 + lb*cos(bth))^2 + m*((l*cos(bth + q1 + q2 + q3))/2 + l*cos(bth + q1) + lb*cos(bth) + l*cos(bth + q1 + q2))^2,                                                                                                                                                                                                                                                                                                                                                                                                                 3*I + Ib;
 -(3*m + mb)*((base_y*mb)/(3*m + mb) - base_y + (m*(3*base_y + (l*sin(bth + q1 + q2 + q3))/2 + (5*l*sin(bth + q1))/2 + 3*lb*sin(bth) + (3*l*sin(bth + q1 + q2))/2))/(3*m + mb)), (3*m + mb)*((base_x*mb)/(3*m + mb) - base_x + (m*(3*base_x + (l*cos(bth + q1 + q2 + q3))/2 + (5*l*cos(bth + q1))/2 + 3*lb*cos(bth) + (3*l*cos(bth + q1 + q2))/2))/(3*m + mb)),                                                                                                                                                                              0,                                                                                                                                                                                                                                                                                                                                                                                         3*I + Ib,                                                                                                                                                                                                                                                                                                                                                                                         3*I + Ib, 3*I + Ib + m*(l*cos(bth + q1) + lb*cos(bth) + (l*cos(bth + q1 + q2))/2)^2 + m*((l*cos(bth + q1))/2 + lb*cos(bth))^2 + m*(l*sin(bth + q1) + lb*sin(bth) + (l*sin(bth + q1 + q2))/2)^2 + m*((l*cos(bth + q1 + q2 + q3))/2 + l*cos(bth + q1) + lb*cos(bth) + l*cos(bth + q1 + q2))^2 + m*((l*sin(bth + q1))/2 + lb*sin(bth))^2 + m*((l*sin(bth + q1 + q2 + q3))/2 + l*sin(bth + q1) + lb*sin(bth) + l*sin(bth + q1 + q2))^2];
 


Hbm=[                                                                                                                                                                                                                                                                                                                                                                                                                                         -m*((l*sin(bth + q1 + q2 + q3))/2 + (5*l*sin(bth + q1))/2 + (3*l*sin(bth + q1 + q2))/2), -m*((l*sin(bth + q1 + q2 + q3))/2 + (3*l*sin(bth + q1 + q2))/2), -(l*m*sin(bth + q1 + q2 + q3))/2;
                                                                                                                                                                                                                                                                                                                                                                                                                                          m*((l*cos(bth + q1 + q2 + q3))/2 + (5*l*cos(bth + q1))/2 + (3*l*cos(bth + q1 + q2))/2),  m*((l*cos(bth + q1 + q2 + q3))/2 + (3*l*cos(bth + q1 + q2))/2),  (l*m*cos(bth + q1 + q2 + q3))/2;
                                                                                                                                                                                                                                                                                                                                                                                                                                                                                                                               0,                                                               0,                                0;
                                                                                                                                                                                                                                                                                                                                                                                                                                                                                                                               0,                                                               0,                                0;
                                                                                                                                                                                                                                                                                                                                                                                                                                                                                                                               0,                                                               0,                                0;
 3*I + (l*m*cos(bth + q1)*((l*cos(bth + q1))/2 + lb*cos(bth)))/2 + (l*m*sin(bth + q1)*(l*sin(bth + q1) + lb*sin(bth) + (l*sin(bth + q1 + q2))/2))/2 + (l*m*cos(bth + q1)*((l*cos(bth + q1 + q2 + q3))/2 + l*cos(bth + q1) + lb*cos(bth) + l*cos(bth + q1 + q2)))/2 + (l*m*sin(bth + q1)*((l*sin(bth + q1))/2 + lb*sin(bth)))/2 + (l*m*sin(bth + q1)*((l*sin(bth + q1 + q2 + q3))/2 + l*sin(bth + q1) + lb*sin(bth) + l*sin(bth + q1 + q2)))/2 + (l*m*cos(bth + q1)*(l*cos(bth + q1) + lb*cos(bth) + (l*cos(bth + q1 + q2))/2))/2,                                                             2*I,                                I];
 





%Jacobian Manipulator
Jm =[ - l*sin(bth + q1 + q2 + q3) - l*sin(bth + q1) - l*sin(bth + q1 + q2), - l*sin(bth + q1 + q2 + q3) - l*sin(bth + q1 + q2), -l*sin(bth + q1 + q2 + q3);
    l*cos(bth + q1 + q2 + q3) + l*cos(bth + q1) + l*cos(bth + q1 + q2),   l*cos(bth + q1 + q2 + q3) + l*cos(bth + q1 + q2),  l*cos(bth + q1 + q2 + q3);
                                                                     0,                                                  0,                          0;
                                                                     0,                                                  0,                          0;
                                                                     0,                                                  0,                          0;
                                                                     0,                                                  0,                          0];
 

SCnew=-inv(Hb)*Hbm*[qd1; qd2; qd3];

%Jacobian Base
Jb =[ 1, 0, 0,                                                                                0,                                                                                  0, - l*sin(bth + q1 + q2 + q3) - l*sin(bth + q1) - lb*sin(bth) - l*sin(bth + q1 + q2);
  0, 1, 0,                                                                                0,                                                                                  0,   l*cos(bth + q1 + q2 + q3) + l*cos(bth + q1) + lb*cos(bth) + l*cos(bth + q1 + q2);
  0, 0, 1, l*sin(bth + q1 + q2 + q3) + l*sin(bth + q1) + lb*sin(bth) + l*sin(bth + q1 + q2), - l*cos(bth + q1 + q2 + q3) - l*cos(bth + q1) - lb*cos(bth) - l*cos(bth + q1 + q2),                                                                                  0;
  0, 0, 0,                                                                                1,                                                                                  0,                                                                                  0;
  0, 0, 0,                                                                                0,                                                                                  1,                                                                                  0;
  0, 0, 0,                                                                                0,                                                                                  0,                                                                                  1];
 

%Generalized Jacobian
Jstar=Jm-Jb*inv(Hb)*Hbm;

EE=[0;0;q3rd];
invJstar=pinv(Jstar);
qd_req=invJstar*Ve+EE;

A=svd(Jstar);
lambmax=20;
Sigma=A(3);
if Sigma>=0.5 
lamb2=0;
else
lamb2=(1-((Sigma)/4)^2)*lambmax;
end
qd_reqW=(Jstar'*pinv(Jstar*Jstar'+(lamb2)*eye(6)))*Ve+EE;

end

== matlab function CusakisME4901delay/Energy Measures/MATLAB Function2 ==
  data: E output; t1 input; t2 input; t3 input; qd1 input; qd2 input; qd3 input; Mem input; Etot output
function [E,Etot]  = fcn(t1,t2,t3,qd1,qd2,qd3,Mem)
%#codegen


a=abs(t1*qd1);

b=abs(t2*qd2);

c=abs(t3*qd3);


E=a+b+c;


Etot=E+Mem;

== matlab function CusakisME4901delay/VR Simulator/MATLAB Function ==
  data: t input; orbit output
function orbit = fcn(t)
%#codegen



w=0.01;

x=cos(w*t);

z=sin(w*t);

y=0;

%orbit = [x;y;z];

orbit = [0;0;0];

== matlab function CusakisME4901delay/Hardware Interface Comuincation/rad to Arm/MATLAB Function1 ==
  data: u input; y output
function y = fcn(u)
%#codegen
udeg=u*180/pi;

%degrees to arduino angles..(avoids negative numbers)
y = (udeg+180)*10;

== matlab function CusakisME4901delay/Differential Kinematics1/Impact mass/Button Selector ==
  data: but input; y output; bo input
function y   = fcn(but,bo)
%#codegen


b=but(4);

if b==1
if bo==0
y=1;
else
y=0;
end
else
if bo==1
y=1;
else
y=0;
end
end

== matlab function CusakisME4901delay/Differential Kinematics1/Impact mass/Force Measure ==
  data: u input; mt parameter; a output; mb parameter; m parameter
function a = fcn(u,mt,mb,m)
%#codegen


% F = M a

r=mt/(mb+3*m);
a=zeros([6,1]); %accelerations on the end effector

a(1)=-r*u(1);
a(2)=-r*u(2);
a(6)=-r*u(3);

== matlab function CusakisME4901delay/Differential Kinematics1/Impact mass/3rd link Kinematics1 ==
  data: Ve input; Vlinkcoll input; Ve_out output
function Ve_out  = fcn(Ve,Vlinkcoll)
%#codegen

%adding the velocities due to the collision

Ve_out=zeros([6,1]);

Ve_out(1)=Ve(1)+Vlinkcoll(1);

Ve_out(2)=Ve(2)+Vlinkcoll(2);

Ve_out(6)=Ve(6)+Vlinkcoll(6);

end

== matlab function CusakisME4901delay/Hardware Interface Comuincation/rad to Arm/MATLAB Function2 ==
  data: u input; y output
function y = fcn(u)
%#codegen
udeg=u*180/pi;

%degrees to arduino angles..(avoids negative numbers)
y = (udeg+180)*10;
